simulink model "SEBPIRD_model"  (R2023a)
settings: Solver=VariableStepAuto  StartTime=0.0  StopTime=365  RelTol=1e-3
values from neighbouring files (symbols this model uses):
  b = 1.2    [parameters_covid.mat]
  delta = 0.002    [parameters_covid.mat]
  g = 0.1    [parameters_covid.mat]
  lambda = 0.166666666667    [parameters_covid.mat]
  N = 7500000    [parameters_covid.mat]
  omega = 0.01    [parameters_covid.mat]
  psi = 0.0025    [parameters_covid.mat]
settings Model: Creator=mluser  LastModifiedBy=mluser

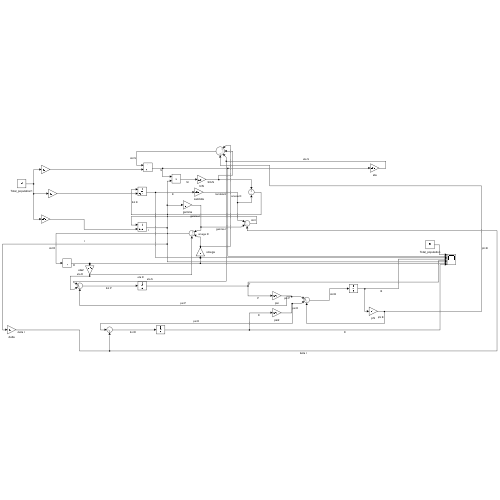
[thumbnail: Simulink's stored preview of the top-level diagram]
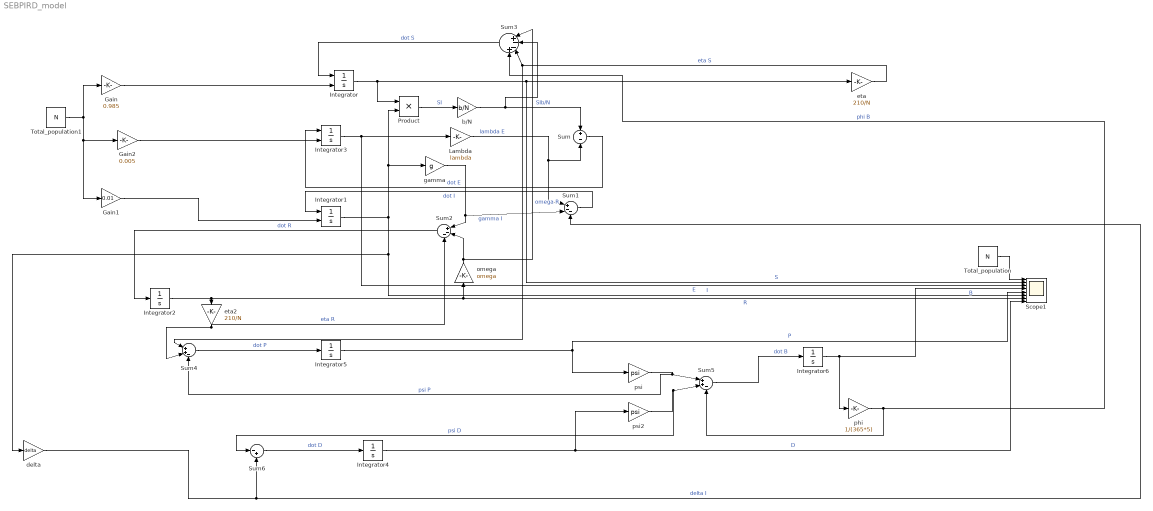
== system SEBPIRD_model ==
  Gain : Gain  Gain=0.985
  Gain1 : Gain  Gain=0.01
  Gain2 : Gain  Gain=0.005
  Integrator : Integrator  InitialConditionSource=external  InitialCondition=N
  Integrator1 : Integrator  InitialConditionSource=external
  Integrator{2,4..6} (4 alike) : Integrator
  Integrator3 : Integrator  InitialConditionSource=external
  Lambda : Gain  Gain=lambda
  Product : Product
  Scope1 : Scope  NumInputPorts=8
  Sum : Sum  Inputs=+-
  Sum1 : Sum  Inputs=|+--
  Sum2 : Sum  Inputs=|+--
  Sum3 : Sum  Inputs=|+--+
  Sum4 : Sum  Inputs=|++-
  Sum5 : Sum  Inputs=|++-
  Sum6 : Sum  Inputs=|-+
  Total_population : Constant  Value=N
  Total_population1 : Constant  Value=N
  b/N : Gain  Gain=b/N
  delta : Gain  Gain=delta
  eta : Gain  Gain=210/N
  eta2 : Gain  Gain=210/N
  gamma : Gain  Gain=g
  omega : Gain  Gain=omega
  phi : Gain  Gain=1/(365*5)
  psi : Gain  Gain=psi
  psi2 : Gain  Gain=psi
  wires:
  Integrator/1 -> Product/1, eta/1, Scope1/2  "S"
  Product/1 -> b/N/1  "SI"
  gamma/1 -> Sum2/1, Sum1/2  "gamma I"
  Sum/1 -> Integrator3/1  "dot E"
  Sum2/1 -> Integrator2/1  "dot R"
  Integrator2/1 -> Scope1/7, omega/1, eta2/1  "R"
  b/N/1 -> Sum/1, Sum3/2  "SIb/N"
  Sum3/1 -> Integrator/1  "dot S"
  Integrator1/1 -> gamma/1, Product/2, delta/1, Scope1/6  "I"
  Gain/1 -> Integrator/2
  Gain1/1 -> Integrator1/2
  Total_population/1 -> Scope1/1
  Integrator3/1 -> Lambda/1, Scope1/3  "E"
  Total_population1/1 -> Gain1/1, Gain2/1, Gain/1
  Gain2/1 -> Integrator3/2
  Lambda/1 -> Sum/2, Sum1/1  "lambda E"
  Sum1/1 -> Integrator1/1  "dot I"
  Integrator4/1 -> psi2/1, Scope1/8  "D"
  omega/1 -> Sum3/1, Sum2/2  "omega R"
  delta/1 -> Sum6/2, Sum1/3  "delta I"
  Integrator5/1 -> Scope1/5, psi/1  "P"
  eta/1 -> Sum4/1, Sum3/3  "eta S"
  Sum4/1 -> Integrator5/1  "dot P"
  eta2/1 -> Sum4/2, Sum2/3  "eta R"
  Integrator6/1 -> phi/1, Scope1/4  "B"
  psi/1 -> Sum4/3, Sum5/1  "psi P"
  psi2/1 -> Sum6/1, Sum5/2  "psi D"
  Sum5/1 -> Integrator6/1  "dot B"
  phi/1 -> Sum3/4, Sum5/3  "phi B"
  Sum6/1 -> Integrator4/1  "dot D"
